simulink model "door_integralAction"  (R2023b)
settings: Solver=VariableStepAuto  StartTime=0.0  StopTime=3  RelTol=1e-3
values from neighbouring files (symbols this model uses):
  A = plant.A    [door.m]
  B = plant.B    [door.m]
  C = [0,0,1]    [door.m]
  F = Kint(1:3)    [door.m]
  H = Kint(4)    [door.m]
settings Model: Creator=demkv  LastModifiedBy=demkv

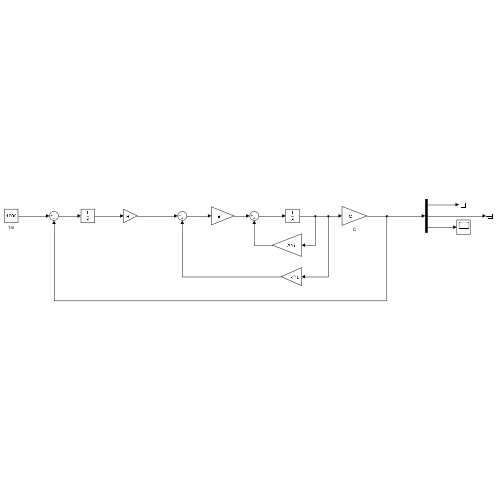
[thumbnail: Simulink's stored preview of the top-level diagram]
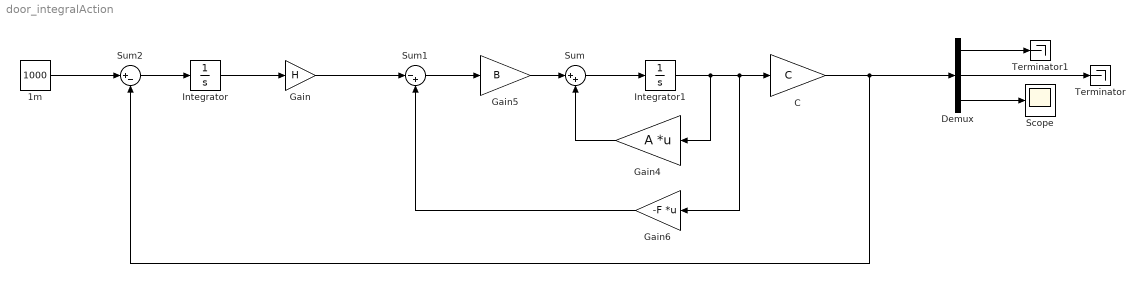
== system door_integralAction ==
  1m : Constant  Value=1000
  C : Gain  Gain=C
  Demux : Demux  Outputs=3
  Gain : Gain  Gain=H
  Gain4 : Gain  Gain=A  Multiplication=Matrix(K*u)
  Gain5 : Gain  Gain=B
  Gain6 : Gain  Gain=-F  Multiplication=Matrix(K*u)
  Integrator : Integrator
  Integrator1 : Integrator
  Scope : Scope
  Sum : Sum  Inputs=|++
  Sum1 : Sum  Inputs=|-+
  Sum2 : Sum  Inputs=|+-
  Terminator : Terminator
  Terminator1 : Terminator
  wires:
  Gain4/1 -> Sum/2
  Sum/1 -> Integrator1/1
  Integrator1/1 -> Gain4/1, Gain6/1, C/1
  Sum1/1 -> Gain5/1
  Gain6/1 -> Sum1/2
  Gain5/1 -> Sum/1
  Gain/1 -> Sum1/1
  Integrator/1 -> Gain/1
  C/1 -> Demux/1, Sum2/2
  Sum2/1 -> Integrator/1
  1m/1 -> Sum2/1
  Demux/2 -> Terminator/1
  Demux/3 -> Scope/1
  Demux/1 -> Terminator1/1
